simulink model "p_controller"  (R2022a)
settings: Solver=VariableStepAuto  StartTime=0.0  StopTime=10.0  RelTol=1e-3
settings Model: Creator=mluser  LastModifiedBy=mluser

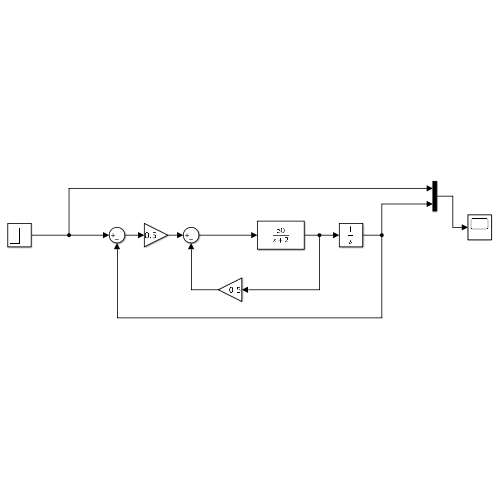
[thumbnail: Simulink's stored preview of the top-level diagram]
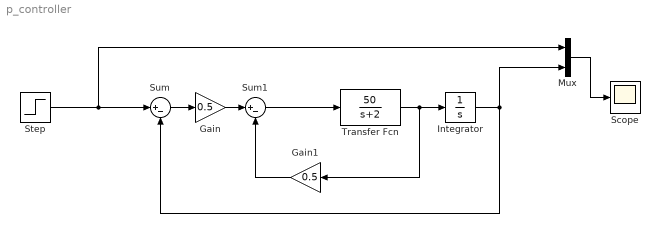
== system p_controller ==
  Gain : Gain  Gain=0.5
  Gain1 : Gain  Gain=0.5
  Integrator : Integrator
  Mux : Mux  Inputs=2
  Scope : Scope
  Step : Step  After=0.5  SampleTime=0
  Sum : Sum  Inputs=|+-
  Sum1 : Sum  Inputs=|+-
  Transfer Fcn : TransferFcn  Numerator=[50]  Denominator=[1 2]
  wires:
  Step/1 -> Mux/1, Sum/1
  Sum1/1 -> Transfer Fcn/1
  Sum/1 -> Gain/1
  Gain/1 -> Sum1/1
  Transfer Fcn/1 -> Gain1/1, Integrator/1
  Mux/1 -> Scope/1
  Integrator/1 -> Sum/2, Mux/2
  Gain1/1 -> Sum1/2
